simulink model "Dan_model1_2"  (Simulink 7.8)
settings: Solver=ode45  StartTime=0.0  StopTime=10.0  RelTol=1e-3
undefined symbols (not defined in the file or in its folder): T
settings Model: Creator=narmada_hm  LastModifiedBy=Dan
settings GRTTargetCC: CombineOutputUpdateFcns=on

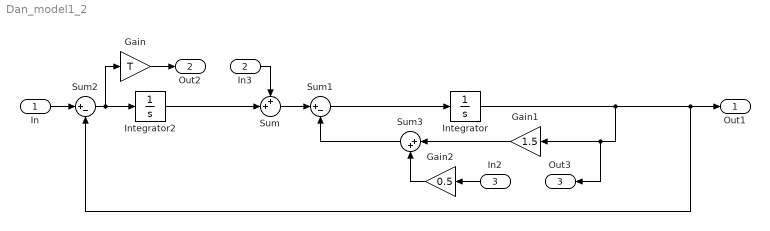
== system Dan_model1_2 ==
  In : Inport
  In3 : Inport  Port=2
  In2 : Inport  Port=3
  Gain : Gain  Gain=T
  Gain1 : Gain  Gain=1.5
  Gain2 : Gain  Gain=0.5
  Integrator : Integrator
  Integrator2 : Integrator
  Sum : Sum  Inputs=++|
  Sum1 : Sum  Inputs=|+-
  Sum2 : Sum  Inputs=|+-
  Sum3 : Sum  Inputs=|++
  Out1 : Outport
  Out2 : Outport  Port=2
  Out3 : Outport  Port=3
  wires:
  Sum1/1 -> Integrator/1
  Gain/1 -> Out2/1
  In/1 -> Sum2/1
  Sum2/1 -> Gain/1, Integrator2/1
  Sum/1 -> Sum1/1
  In2/1 -> Gain2/1
  Gain1/1 -> Sum3/1
  Sum3/1 -> Sum1/2
  Gain2/1 -> Sum3/2
  In3/1 -> Sum/1
  Integrator2/1 -> Sum/2
  Integrator/1 -> Gain1/1, Out3/1, Sum2/2, Out1/1
